simulink model "OCTModel"  (R2022a)
settings: Solver=ode23tb  StartTime=0.0  StopTime=simParams.duration.Value  FixedStep=0.1  MaxStep=sqrt(simParams.lengthScaleFactor.Value)  RelTol=1e-3  AbsTol=1e-3
undefined symbols (not defined in the file): hiLvlController, HILVLCONTROLLER, hiLvlController_cl, initializeVariantsFromBlock, plant, PLANT, plant_cl
libraries: environment_cl x1, flightController_cl x1, gndStnController_cl x1, FSHiLvl_cl x1, constantBasisParameters_cl x1, gpkfAltitudeOpt_cl x1, gpkfPathOpt_cl x1, gpkfPathOptWithRGPinnerLoop_cl x1, ilcPathOpt_cl x1, ilcPathOptThrTen_cl x1, variableAltitudeBasisParams_cl x1, variableRadiusBasisParams_cl x1
PreSaveFcn:
  | % Callback to reset the view so that the
  | % the next person to open isn't totally lost.
  | hilite_system('OCTModel/plant');
  | hilite_system('OCTModel/plant','none');
  | set_param(gcs,'Zoomfactor','fit to view')
settings Model: SimulationMode=accelerator  PauseTimes=49.09  PacingRate=1000  ExtModeTrigDuration=100  Creator=mcobb  LastModifiedBy=benjiwu
settings SolverCC: AlgebraicLoopSolver=LineSearch  SolverResetMethod=Robust  MinimalZcImpactIntegration=on
settings DataIOCC: SaveOperatingPoint=on  SaveFormat=Array  SaveOutput=off  DSMLogging=off  ReturnWorkspaceOutputs=off  StateSaveName=tmp_raccel_xout
settings OptimizationCC: DefaultParameterBehavior=Inlined  EnhancedBackFolding=on  PassReuseOutputArgsThreshold=0  EfficientMapNaN2IntZero=off  OptimizeBlockOrder=speed  DifferentSizesBufferReuse=on  OptimizationCustomize=off
settings DebuggingCC: SignalRangeChecking=error  AlgebraicLoopMsg=none  ArtificialAlgebraicLoopMsg=none  ParameterTunabilityLossMsg=error  UnconnectedInputMsg=warning  UnconnectedOutputMsg=warning  UnconnectedLineMsg=warning  BusObjectLabelMismatch=error  SFMachineParentedDataDiag=warning  ArithmeticOperatorsInVariantConditions=warning
settings HardwareCC: TargetBitPerLong=64  TargetBitPerPointer=64  TargetBitPerSizeT=64  TargetBitPerPtrDiffT=64  TargetLongLongMode=on  TargetIntDivRoundTo=Zero  TargetEndianess=LittleEndian  TargetWordSize=64  TargetHWDeviceType=MATLAB Host  ProdEqTarget=off
settings SFSimCC: MATLABDynamicMemAlloc=off  CustomCodeUndefinedFunction=UseInterfaceOnly
settings CodeAppCC: MaxIdLength=128
settings GRTTargetCC: CombineOutputUpdateFcns=off  GRTInterface=on

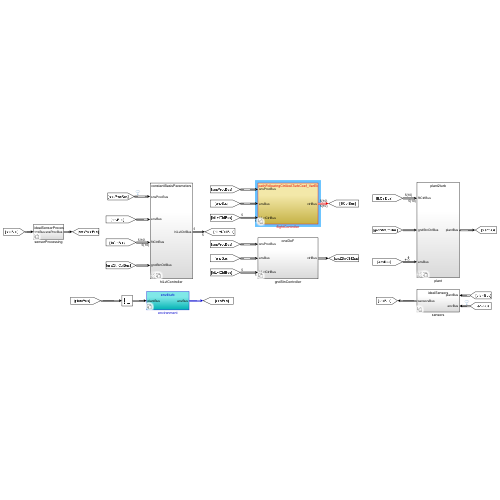
[thumbnail: Simulink's stored preview of the top-level diagram]
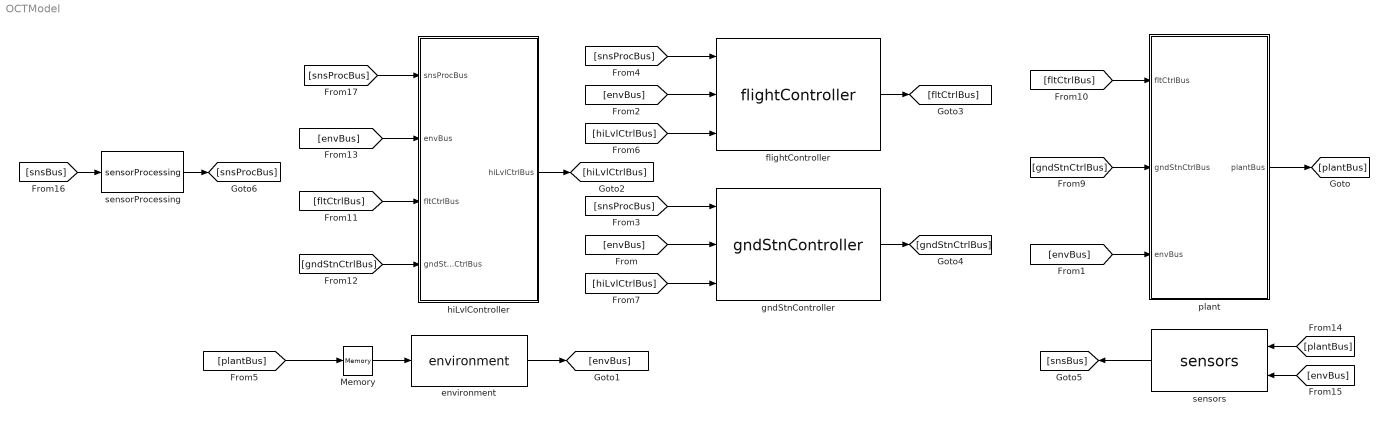
== system OCTModel ==
  Memory : Memory
  environment : environment_cl/environment  SystemSampleTime=-1  VariantActivationTime=update diagram  Latency=0  AutoFrameSizeCalculation=off
  flightController : flightController_cl/flightController  SystemSampleTime=-1  VariantActivationTime=update diagram  Latency=0  AutoFrameSizeCalculation=off
      link override FSCtrlDtrVhcl/Compare To Constant2: const=2
      link override FSCtrlDtrVhcl/Gain2: Gain=0.55
      link override FSCtrlDtrVhcl/non-xcurrent/LaRController/Pitch Setpoint Control/filteredPIDControllerAW: cmax=LaRCtrl.pitchAngleMax.upperLimit.Value  cmin=LaRCtrl.pitchAngleMax.lowerLimit.Value
      link override FSCtrlDtrVhcl/non-xcurrent/LaRController/pitchFlag1: Value=pthCtrl1.RPMConst.Value*ones(vhcl.numTurbines.Value,1)
      link override FSCtrlDtrVhcl/xcurrent-lemOfBooth1/pathFollowingCtrlAoATurb: pathCtrl=pthCtrl1
      link override FSCtrlDtrVhcl/xcurrent-lemOfBooth1/pathFollowingCtrlAoATurb/Constant2: Value=pathCtrl.RPMConst.Value*ones(vhcl.numTurbines.Value,1)
      link override pathFollowingCtrlAoATurb/Constant4: Value=2
      link override pathFollowingCtrlAoATurb/Cp look-up1: BreakpointsForDimension1=vhcl.turb1.RPMref.Value  Table=vhcl.turb1.CtLookup.Value
      link override pathFollowingCtrlAoATurb/From46: GotoTag=velWindBdy
      link override pathFollowingCtrlAoATurb/From68: GotoTag=dragVec
      link override pathFollowingCtrlAoATurb/Gain2: Gain=.5
      link override pathFollowingCtrlAoATurb/Gain3: Gain=180/pi
      link override pathFollowingCtrlAoATurb/Switch1: Threshold=1e6
      link override pathFollowingCtrlAoATurb/courseFollowLookAhead/Constant: Value=0
      link override pathFollowingCtrlAoATurb/desiredMoment1/Ramp: InitialOutput=1
      link override pathFollowingCtrlAoATurb/desiredMoment1/Sine Wave: TimeSource=Use external signal  Amplitude=3*pi/180  Bias=25*pi/180  Frequency=4*pi  Phase=pi/2
      link override pathFollowingCtrlAoATurb/fluidDynamicSurface: vcl=vhcl  fluidMomentArms=vhcl.fluidMomentArms.Value  fluidRefArea=vhcl.fluidRefArea.Value  wingTips=vhcl.wingTipPositions.Value
      link override pathFollowingCtrlAoATurb/rotorTorqueCtrl: rho=fluidDensity
      link override pathFollowingCtrlAoATurbCoef: pathCtrl=fltCtrl
      link override pathFollowingCtrlAoATurbCoef/Saturation: UpperLimit=90  LowerLimit=-90
      link override pathFollowingCtrlAoATurbCoef/desiredMoment1/Constant9: Value=[2 2 2]
      link override pathFollowingCtrlAoATurbCoef/desiredMoment1/Goto17: GotoTag=velMag
      link override pathFollowingCtrlAoATurbCoef/desiredMoment1/Ramp: InitialOutput=0.2  slope=0.01  start=200
      link override pathFollowingCtrlAoATurbCoef/desiredMoment1/Ramp1: InitialOutput=1
      link override pathFollowingCtrlAoATurbCoef/desiredMoment1/Sine Wave: Amplitude=2*pi/180  Bias=12*pi/180
      link override pathFollowingCtrlAoATurbCoef/rotorTorqueCtrl/Coefficient of torque lookup2: BreakpointsForDimension1=turb_struct.tauCoefTSR(end:-1:1)  Table=turb_struct.tauCoefLookup(end:-1:1)
      link override pathFollowingCtrlAoATurbCoef/rotorTorqueCtrl/Constant25: Value=pi*(turb_struct.diameter/2)^3
      link override pathFollowingCtrlAoATurbCoef_VarElvAzu: pathCtrl=fltCtrl
      link override pathFollowingCtrlAoATurbCoef_VarElvAzu/temp_ElvAzuSP/Rate Limiter: RisingSlewLimit=0.025*pi/180  FallingSlewLimit=-0.025*pi/180
      link override pathFollowingCtrlAoATurbCoef_VarElvAzu/temp_ElvAzuSP/Rate Limiter1: RisingSlewLimit=flwSpd/2  FallingSlewLimit=-flwSpd/2
      link override pathFollowingCtrlAoATurbOpt: pathCtrl=fltCtrl
      link override pathFollowingCtrlAoATurbOpt/Goto13: GotoTag=vAppBdy
      link override pathFollowingCtrlAoATurbOpt/Pulse Generator: TimeSource=Use external signal  Period=5
      link override pathFollowingCtrlAoATurbOpt/Switch1: Threshold=30
      link override pathFollowingCtrlAoATurbOpt/courseFollowLookAhead/Constant: Value=0
      link override pathFollowingCtrlAoATurbOpt/desiredMoment1/Sine Wave: Bias=30*pi/180
      link override pathFollowingCtrlAoATurbOpt/rotorTorqueCtrl1: rho=fluidDensity
      link override pathFollowingCtrlAoATurbOpt/rotorTorqueCtrl1/Gain: Gain=20
      link override scaleTest/manta38TestCampaign/orientation/pathFollowingCtrlAoATurbCoefDiscrete/Gain: Gain=[1 1 1 1]
  gndStnController : gndStnController_cl/gndStnController  SystemSampleTime=-1  VariantActivationTime=update diagram  Latency=0  AutoFrameSizeCalculation=off
  hiLvlController : Subsystem  AncestorBlock=hiLvlController_cl/hiLvlController  LoadFcn=initializeVariantsFromBlock(gcb)  InitFcn=initializeVariantsFromBlock(gcb)  StartFcn=initializeVariantsFromBlock(gcb)  Variant=on
  plant : Subsystem  AncestorBlock=plant_cl/plant  Variant=on
  sensorProcessing : sensorProcessing_cl/sensorProcessing  SystemSampleTime=-1  VariantActivationTime=update diagram  Latency=0  AutoFrameSizeCalculation=off
  sensors : sensors_cl/sensors  SystemSampleTime=-1  VariantActivationTime=update diagram  Latency=0  AutoFrameSizeCalculation=off
  wires:
  Memory/1 -> environment/1
  [envBus] -> gndStnController/2
  [snsProcBus] -> gndStnController/1
  [snsProcBus] -> hiLvlController/1(snsProcBus)
  flightController/1 -> [fltCtrlBus]
  gndStnController/1 -> [gndStnCtrlBus]
  [envBus] -> hiLvlController/2(envBus)
  [fltCtrlBus] -> hiLvlController/3(fltCtrlBus)
  [gndStnCtrlBus] -> hiLvlController/4(gndStnCtrlBus)
  [plantBus] -> Memory/1
  [hiLvlCtrlBus] -> flightController/3
  [hiLvlCtrlBus] -> gndStnController/3
  hiLvlController/1(hiLvlCtrlBus) -> [hiLvlCtrlBus]
  [envBus] -> flightController/2
  [plantBus] -> sensors/1
  [envBus] -> sensors/2
  sensors/1 -> [snsBus]
  [snsBus] -> sensorProcessing/1
  sensorProcessing/1 -> [snsProcBus]
  plant/1(plantBus) -> [plantBus]
  [fltCtrlBus] -> plant/1(fltCtrlBus)
  [gndStnCtrlBus] -> plant/2(gndStnCtrlBus)
  [envBus] -> plant/3(envBus)
  environment/1 -> [envBus]
  [snsProcBus] -> flightController/1

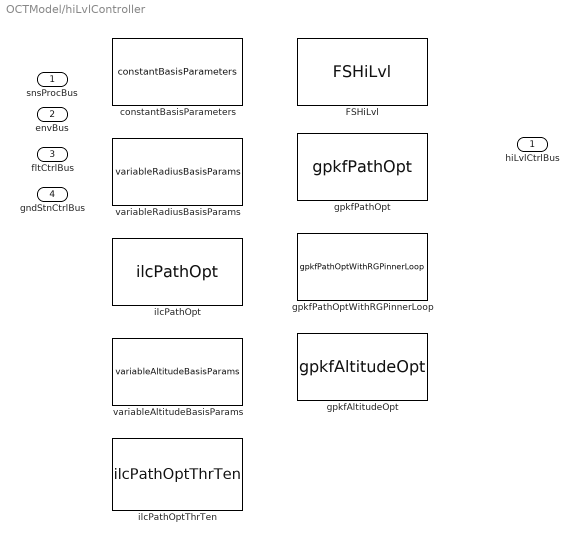
== system OCTModel/hiLvlController ==
  snsProcBus : Inport  OutDataTypeStr=Bus: sensorsProcessingBus
  envBus : Inport  Port=2  OutDataTypeStr=Bus: envBus
  fltCtrlBus : Inport  Port=3  OutDataTypeStr=Bus: fltCtrlBus
  gndStnCtrlBus : Inport  Port=4  OutDataTypeStr=Bus: gndStnCtrlBus
  FSHiLvl : FSHiLvl_cl/FSHiLvl  VariantControl=strcmpi(HILVLCONTROLLER,'mantaFSHiLvl')  hiLvlCtrl=hiLvlCtrl
  constantBasisParameters : constantBasisParameters_cl/constantBasisParameters  VariantControl=strcmpi(HILVLCONTROLLER,'constantBasisParameters')  hiLvlCtrl=hiLvlCtrl
  gpkfAltitudeOpt : gpkfAltitudeOpt_cl/gpkfAltitudeOpt  VariantControl=(default)  hiLvlCtrl=hiLvlCtrl
  gpkfPathOpt : gpkfPathOpt_cl/gpkfPathOpt  VariantControl=strcmpi(HILVLCONTROLLER,'gpkfPathOpt')  hiLvlCtrl=hiLvlCtrl
  gpkfPathOptWithRGPinnerLoop : gpkfPathOptWithRGPinnerLoop_cl/gpkfPathOptWithRGPinnerLoop  VariantControl=strcmpi(HILVLCONTROLLER,'gpkfPathOptWithRGPinnerLoop')  hiLvlCtrl=hiLvlCtrl
  ilcPathOpt : ilcPathOpt_cl/ilcPathOpt  VariantControl=strcmpi(HILVLCONTROLLER,'ilcPathOpt')  ctrl=hiLvlCtrl
  ilcPathOptThrTen : ilcPathOptThrTen_cl/ilcPathOptThrTen  VariantControl=strcmpi(HILVLCONTROLLER,'ilcPathOptThrTen')  ctrl=hiLvlCtrl
      link override Compare To Constant2: const=50
      link override From27: GotoTag=basisParams
      link override Variant Subsystem/rotorAoA: VariantControl=sum(hiLvlCtrl.subspaceDims)>12
      link override Variant Subsystem/rotorOptimization: VariantControl=length(fieldnames(hiLvlCtrl.parameterSpace))==1
      link override Variant Subsystem/seILC: VariantControl=(default)
      link override ilcUpdate1: initBasisParams=[ctrl.initBasisParams.Value]  trstRgn=[ctrl.trustRegion.Value]  amp=[ctrl.excitationAmp.Value]  enableVec=[ctrl.optEnable.Value]
      link override ilcUpdate1/Unit Delay: InitialCondition=[initBasisParams(logical(enableVec))]'
      link override pathIteration/Unit Delay: InitialCondition=[initBasisParams(logical(enableVec))]'
      link override switchingILC: trust=.05*[ones(1,12)]  amp=.001*[ones(1,12)]  initBasisParams=[hiLvlCtrl.initBasisParams.Value(1:2) 2.88*ones(1,10)]  lrn=.0005
      link override switchingILC/basisVec: InitialOutput=hiLvlCtrl.initParameters
      link override switchingILC1: initBasisParams=[1 1 2.88*ones(1,10)]  amp=[.02*ones(1,12)]
      link override switchingILC1/Unit Delay3: InitialCondition=initBasisParams'
      link override switchingILC1/Unit Delay5: InitialCondition=lrn
  variableAltitudeBasisParams : variableAltitudeBasisParams_cl/variableAltitudeBasisParams  VariantControl=strcmpi(HILVLCONTROLLER,'variableAltitudeBasisParams')  basisParams=hiLvlCtrl.basisParams.Value
  variableRadiusBasisParams : variableRadiusBasisParams_cl/variableRadiusBasisParams  VariantControl=strcmpi(HILVLCONTROLLER,'variableRadiusBasisParams')  basisParams=hiLvlCtrl.basisParams.Value
  hiLvlCtrlBus : Outport  OutDataTypeStr=Bus: hiLvlCtrlBus  VectorParamsAs1DForOutWhenUnconnected=off

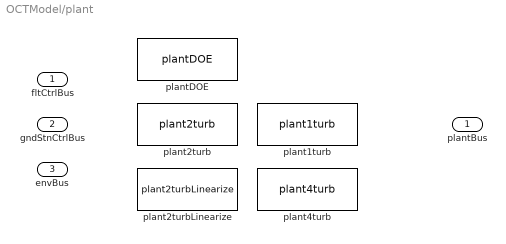
== system OCTModel/plant ==
  fltCtrlBus : Inport
  gndStnCtrlBus : Inport  Port=2
  envBus : Inport  Port=3
  plant1turb : plant1turb_cl/plant1turb  SystemSampleTime=-1  VariantControl=strcmpi(PLANT,'plant1turb')  VariantActivationTime=update diagram  Latency=0  AutoFrameSizeCalculation=off
  plant2turb : plant2turb_cl/plant2turb  SystemSampleTime=-1  VariantControl=strcmpi(PLANT,'plant2turb')  VariantActivationTime=update diagram  Latency=0  AutoFrameSizeCalculation=off
      link override vehicle/vhcl4turb/fuselage/CDFuse: VariantControl=(default)
      link override vehicle/vhcl4turb/fuselage/projAreaFuse: VariantControl=isempty(vhcl.fuse.CD.Value)
  plant2turbLinearize : plant2turbLinearize_cl/plant2turbLinearize  SystemSampleTime=-1  VariantControl=strcmpi(PLANT,'plant2turbLinearize')  VariantActivationTime=update diagram  Latency=0  AutoFrameSizeCalculation=off
  plant4turb : plant4turb_cl/plant4turb  SystemSampleTime=-1  VariantControl=strcmpi(PLANT,'plant4turb')  VariantActivationTime=update diagram  Latency=0  AutoFrameSizeCalculation=off
  plantDOE : plantDOE_cl/plantDOE  SystemSampleTime=-1  VariantControl=strcmpi(PLANT,'plantDOE')  VariantActivationTime=update diagram  Latency=0  AutoFrameSizeCalculation=off
  plantBus : Outport
